simulink model "Structural_11"  (R2022b)
settings: Solver=FixedStepDiscrete  StartTime=0.0  StopTime=1  FixedStep=1  RelTol=1e-3
values from neighbouring files (symbols this model uses):
  E = input('Enter the Value of Youngs Modulus ')    [Test1.m]
  I = input('Enter the Moment of Inertia ')    [Test1.m]
  L = input('Enter the Length of the Wing ')    [Test1.m]
settings Model: Creator=horty  LastModifiedBy=horty

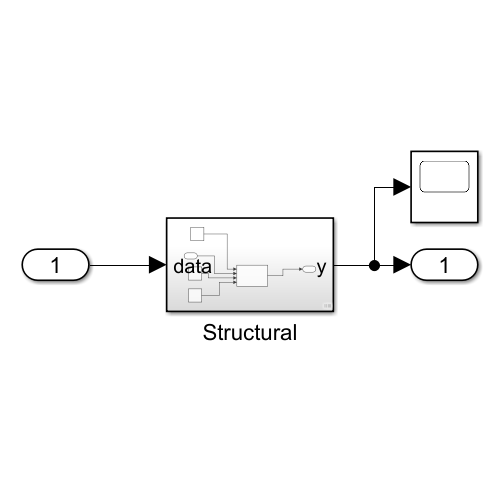
[thumbnail: Simulink's stored preview of the top-level diagram]
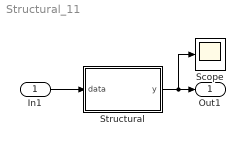
== system Structural_11 ==
  In1 : Inport
  Scope : Scope
  Structural : Subsystem
  Out1 : Outport
  wires:
  Structural/1(y) -> Out1/1, Scope/1
  In1/1 -> Structural/1(data)

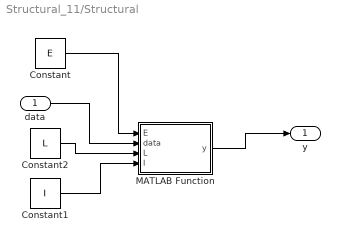
== system Structural_11/Structural ==
  data : Inport
  Constant : Constant  Value=E
  Constant1 : Constant  Value=I
  Constant2 : Constant  Value=L
  MATLAB Function : MATLAB Function  TreatAsAtomicUnit=on
  y : Outport
  wires:
  Constant/1 -> MATLAB Function/1(E)
  MATLAB Function/1(y) -> y/1
  data/1 -> MATLAB Function/2(data)
  Constant2/1 -> MATLAB Function/3(L)
  Constant1/1 -> MATLAB Function/4(I)

== matlab function Structural_11/Structural/MATLAB Function ==
  data: E input; data input; L input; I input; y output
function y = fcn(E, data, L, I)

data=1;
Lift_F=50;
y=Lift_F*(L^3)/(3*E*I);
